simulink model "multichannel_creater"  (R2017b)
settings: Solver=FixedStepDiscrete  StartTime=0.0  StopTime=60  RelTol=1e-3  EnableMultiTasking=on
model workspace (MAT data in the model file):
  MCOS : class17 (value not decoded)
  heli = [0 -3.0517578125e-05 -0.0001220703125 -0.000244140625 -0.0003662109375 -0.000701904296875 -0.00106811523438 -0.00204467773438 -0.00341796875 -0.00460815429688 -0.00595092773438 -0.00762939453125 ... (263304 elements, 263304x1)]
libraries: dspvision x4, dspindex x2
(part 2 of 2)

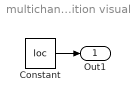
== system multichannel_creater/ Set position visually ==
  Constant : Constant  Value=loc  VectorParams1D=off  SampleTime=-1
  Out1 : Outport
  wires:
  Constant/1 -> Out1/1
